simulink model "nonlinear_model_for_testing_params"  (R2016b)
settings: Solver=VariableStepAuto  StartTime=0.0  StopTime=20  RelTol=1e-3
values from neighbouring files (symbols this model uses):
  B_e = [[0 0] ... (first row only)    [init_heli_all.m]
  j_e = m_c*(l_c)^2 + 2*m_p*(l_h)^2    (= 1.033536)    [init_heli_all.m]
  j_lambda = m_c*(l_c)^2 + 2*m_p*((l_h)^2 + (l_p)^2)    (= 1.077636)    [init_heli_all.m]
  j_p = 2*m_p*(l_p)^2    (= 0.0441)    [init_heli_all.m]
  K = lqr(A, B, Q, R)    [init_heli_all.m]
  L = place(A_e',C_e',[-3,-4,-5,-7,-8,-10]).'    [init_heli_all.m]
  L1 = l_h*k_f    (= 0.10164)    [init_heli_all.m]
  L2 = k2*j_e    (= 0.10164)    [init_heli_all.m]
  L3 = l_h*k_f    (= 0.10164)    [init_heli_all.m]
  L4 = k_f*l_h*l_p    (= 0.017787)    [init_heli_all.m]
  P = inv(C*inv(B*K-A)*B)    [init_heli_all.m]
undefined symbols (not defined in the file or in its folder): A_est
settings Model: Creator=Kevin K. Kaldvansvik  LastModifiedBy=Kevin K. Kaldvansvik

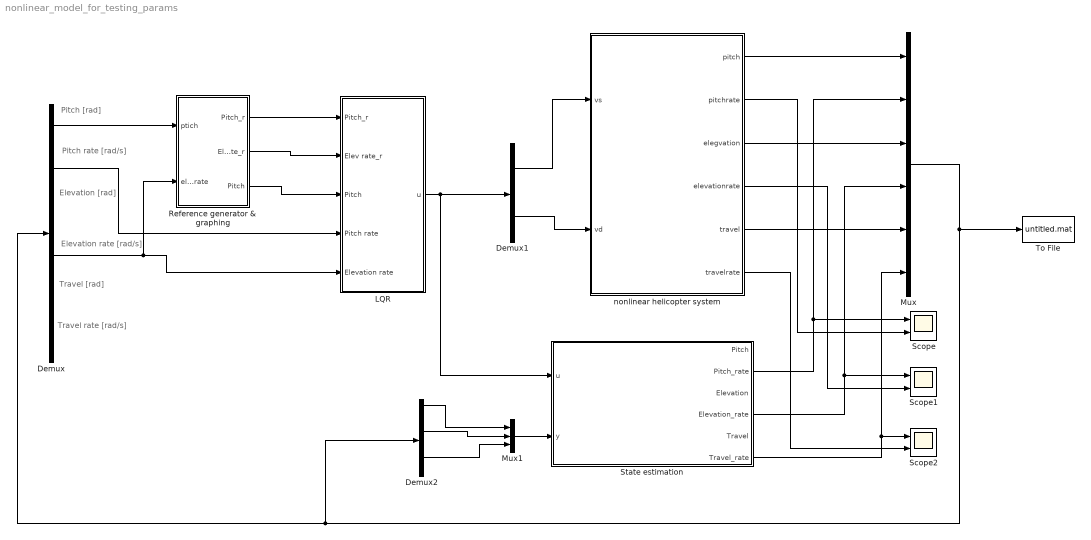
== system nonlinear_model_for_testing_params ==
  note: Travel rate [rad/s]
  note: Travel [rad]
  note: Elevation rate [rad/s]
  note: Elevation [rad]
  note: Pitch rate [rad/s]
  note: Pitch [rad]
  Demux : Demux  Outputs=6
  Demux1 : Demux  Outputs=2
  Demux2 : Demux  Outputs=6
  LQR : Subsystem
  Mux : Mux  Inputs=6
  Mux1 : Mux  Inputs=3
  Reference generator & graphing : Subsystem
  Scope : Scope  NumInputPorts=2
  Scope1 : Scope  NumInputPorts=2
  Scope2 : Scope  NumInputPorts=2
  State estimation : Subsystem
  To File : ToFile  MatrixName=kp_v1
  nonlinear helicopter system : Subsystem
  wires:
  Mux/1 -> Demux2/1, Demux/1, To File/1
  LQR/1(u) -> State estimation/1(u), Demux1/1
  Demux1/1 -> nonlinear helicopter system/1(vs)
  Demux1/2 -> nonlinear helicopter system/2(vd)
  Reference generator & graphing/1(Pitch_r) -> LQR/1(Pitch_r)
  Reference generator & graphing/2(Elevation_rate_r) -> LQR/2(Elev rate_r)
  Reference generator & graphing/3(Pitch) -> LQR/3(Pitch)
  nonlinear helicopter system/1(pitch) -> Mux/1
  nonlinear helicopter system/5(travel) -> Mux/5
  nonlinear helicopter system/3(elegvation) -> Mux/3
  State estimation/4(Elevation_rate) -> Scope1/1, Mux/4
  State estimation/6(Travel_rate) -> Scope2/1, Mux/6
  Demux/1 -> Reference generator & graphing/1(ptich)
  Demux/2 -> LQR/4(Pitch rate)
  Demux/4 -> Reference generator & graphing/2(elevrate), LQR/5(Elevation rate)
  Mux1/1 -> State estimation/2(y)
  Demux2/1 -> Mux1/1
  Demux2/3 -> Mux1/2
  Demux2/5 -> Mux1/3
  State estimation/2(Pitch_rate) -> Scope/1, Mux/2
  nonlinear helicopter system/2(pitchrate) -> Scope/2
  nonlinear helicopter system/4(elevationrate) -> Scope1/2
  nonlinear helicopter system/6(travelrate) -> Scope2/2

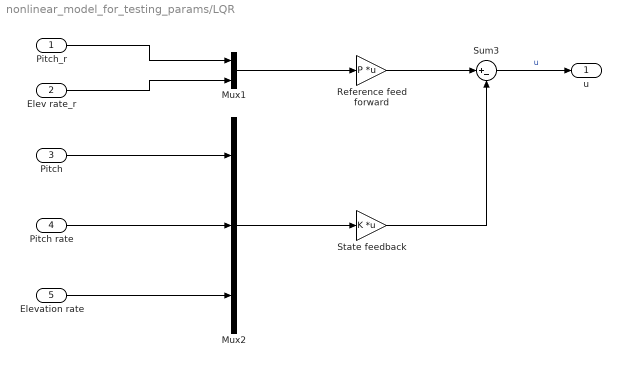
== system nonlinear_model_for_testing_params/LQR ==
  Pitch_r : Inport
  Elev rate_r : Inport  Port=2
  Pitch : Inport  Port=3
  Pitch rate : Inport  Port=4
  Elevation rate : Inport  Port=5
  Mux1 : Mux  Inputs=2
  Mux2 : Mux  Inputs=3
  "Reference feed forward " : Gain  Gain=P  Multiplication=Matrix(K*u)
  State feedback : Gain  Gain=K  Multiplication=Matrix(K*u)
  Sum3 : Sum  Inputs=|+-
  u : Outport
  wires:
  State feedback/1 -> Sum3/2
  "Reference feed forward "/1 -> Sum3/1
  Mux2/1 -> State feedback/1
  Mux1/1 -> "Reference feed forward "/1
  Sum3/1 -> u/1  "u"
  Elev rate_r/1 -> Mux1/2
  Pitch_r/1 -> Mux1/1
  Pitch/1 -> Mux2/1
  Pitch rate/1 -> Mux2/2
  Elevation rate/1 -> Mux2/3

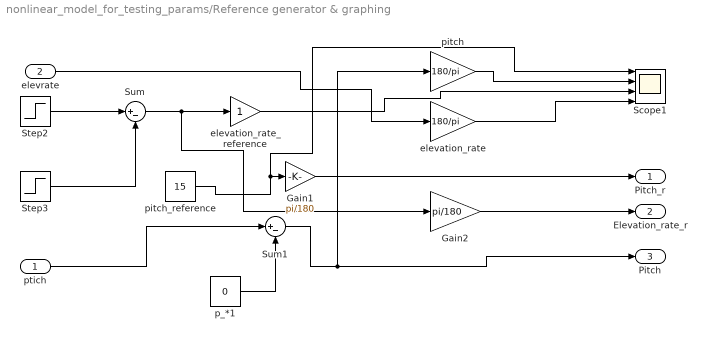
== system nonlinear_model_for_testing_params/Reference generator & graphing ==
  ptich : Inport
  elevrate : Inport  Port=2
  Gain1 : Gain  Gain=pi/180
  Gain2 : Gain  Gain=pi/180
  Scope1 : Scope  NumInputPorts=4
  Step2 : Step  After=5  SampleTime=0
  Step3 : Step  Time=4  After=5  SampleTime=0
  Sum : Sum  Inputs=|+-
  Sum1 : Sum  Inputs=|+-
  elevation_rate : Gain  Gain=180/pi
  elevation_rate_reference : Gain
  p_*1 : Constant  Value=0
  pitch : Gain  Gain=180/pi
  pitch_reference : Constant  Value=15
  Pitch_r : Outport
  Elevation_rate_r : Outport  Port=2
  Pitch : Outport  Port=3
  wires:
  Step3/1 -> Sum/2
  ptich/1 -> Sum1/1
  p_*1/1 -> Sum1/2
  Sum1/1 -> Pitch/1, pitch/1
  Step2/1 -> Sum/1
  Gain1/1 -> Pitch_r/1
  pitch_reference/1 -> Scope1/1, Gain1/1
  Sum/1 -> Gain2/1, elevation_rate_reference/1
  elevation_rate_reference/1 -> Scope1/3
  elevation_rate/1 -> Scope1/4
  pitch/1 -> Scope1/2
  Gain2/1 -> Elevation_rate_r/1
  elevrate/1 -> elevation_rate/1

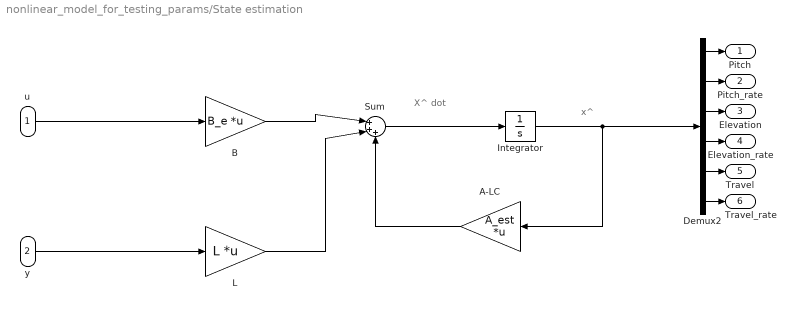
== system nonlinear_model_for_testing_params/State estimation ==
  note: x^
  note: X^ dot
  u : Inport
  y : Inport  Port=2
  A-LC : Gain  Gain=A_est  Multiplication=Matrix(K*u)
  B : Gain  Gain=B_e  Multiplication=Matrix(K*u)
  Demux2 : Demux  Outputs=6
  Integrator : Integrator
  L : Gain  Gain=L  Multiplication=Matrix(K*u)
  Sum : Sum  Inputs=|+++
  Pitch : Outport
  Pitch_rate : Outport  Port=2
  Elevation : Outport  Port=3
  Elevation_rate : Outport  Port=4
  Travel : Outport  Port=5
  Travel_rate : Outport  Port=6
  wires:
  B/1 -> Sum/1
  Sum/1 -> Integrator/1
  Integrator/1 -> A-LC/1, Demux2/1
  L/1 -> Sum/2
  A-LC/1 -> Sum/3
  Demux2/2 -> Pitch_rate/1
  Demux2/3 -> Elevation/1
  Demux2/4 -> Elevation_rate/1
  Demux2/5 -> Travel/1
  Demux2/1 -> Pitch/1
  u/1 -> B/1
  Demux2/6 -> Travel_rate/1
  y/1 -> L/1

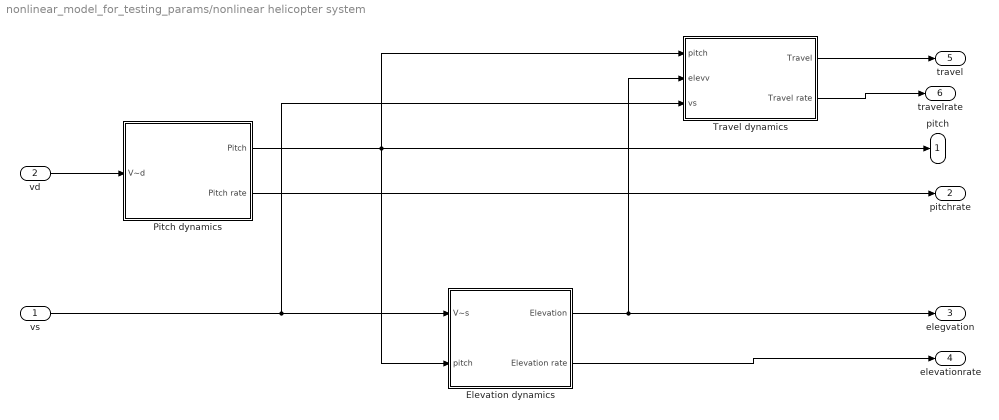
== system nonlinear_model_for_testing_params/nonlinear helicopter system ==
  vs : Inport
  vd : Inport  Port=2
  Elevation dynamics : Subsystem
  Pitch dynamics : Subsystem
  Travel dynamics : Subsystem
  pitch : Outport
  pitchrate : Outport  Port=2
  elegvation : Outport  Port=3
  elevationrate : Outport  Port=4
  travel : Outport  Port=5
  travelrate : Outport  Port=6
  wires:
  vd/1 -> Pitch dynamics/1(V~d)
  Elevation dynamics/1(Elevation) -> Travel dynamics/2(elevv), elegvation/1
  Pitch dynamics/2(Pitch rate) -> pitchrate/1
  vs/1 -> Elevation dynamics/1(V~s), Travel dynamics/3(vs)
  Pitch dynamics/1(Pitch) -> Elevation dynamics/2(pitch), Travel dynamics/1(pitch), pitch/1
  Travel dynamics/2(Travel rate) -> travelrate/1
  Travel dynamics/1(Travel) -> travel/1
  Elevation dynamics/2(Elevation rate) -> elevationrate/1

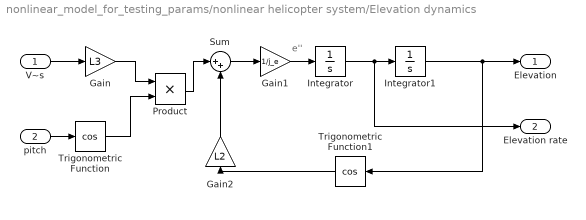
== system nonlinear_model_for_testing_params/nonlinear helicopter system/Elevation dynamics ==
  note: e''
  V~s : Inport
  pitch : Inport  Port=2
  Gain : Gain  Gain=L3
  Gain1 : Gain  Gain=1/j_e
  Gain2 : Gain  Gain=L2
  Integrator : Integrator
  Integrator1 : Integrator
  Product : Product
  Sum : Sum  Inputs=|++
  Trigonometric Function : Trigonometry  Operator=cos
  Trigonometric Function1 : Trigonometry  Operator=cos
  Elevation : Outport
  Elevation rate : Outport  Port=2
  wires:
  Integrator/1 -> Elevation rate/1, Integrator1/1
  V~s/1 -> Gain/1
  Integrator1/1 -> Trigonometric Function1/1, Elevation/1
  Gain/1 -> Product/1
  Sum/1 -> Gain1/1
  Gain1/1 -> Integrator/1
  Product/1 -> Sum/1
  pitch/1 -> Trigonometric Function/1
  Trigonometric Function/1 -> Product/2
  Trigonometric Function1/1 -> Gain2/1
  Gain2/1 -> Sum/2

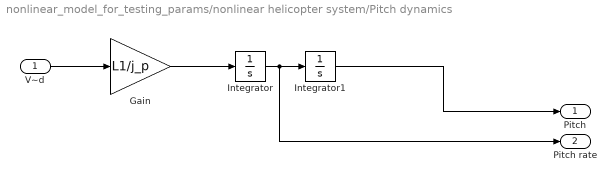
== system nonlinear_model_for_testing_params/nonlinear helicopter system/Pitch dynamics ==
  V~d : Inport
  Gain : Gain  Gain=L1/j_p
  Integrator : Integrator
  Integrator1 : Integrator
  Pitch : Outport
  Pitch rate : Outport  Port=2
  wires:
  Integrator/1 -> Pitch rate/1, Integrator1/1
  Integrator1/1 -> Pitch/1
  V~d/1 -> Gain/1
  Gain/1 -> Integrator/1

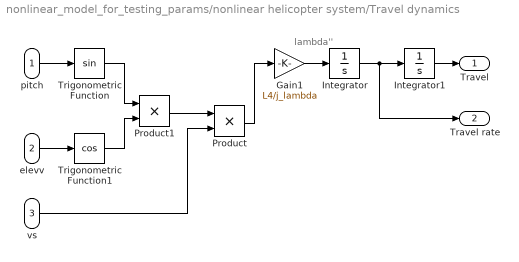
== system nonlinear_model_for_testing_params/nonlinear helicopter system/Travel dynamics ==
  note: lambda''
  pitch : Inport
  elevv : Inport  Port=2
  vs : Inport  Port=3
  Gain1 : Gain  Gain=L4/j_lambda
  Integrator : Integrator
  Integrator1 : Integrator
  Product : Product
  Product1 : Product
  Trigonometric Function : Trigonometry
  Trigonometric Function1 : Trigonometry  Operator=cos
  Travel : Outport
  Travel rate : Outport  Port=2
  wires:
  Integrator1/1 -> Travel/1
  Integrator/1 -> Integrator1/1, Travel rate/1
  pitch/1 -> Trigonometric Function/1
  Gain1/1 -> Integrator/1
  elevv/1 -> Trigonometric Function1/1
  Product/1 -> Gain1/1
  Trigonometric Function/1 -> Product1/1
  Trigonometric Function1/1 -> Product1/2
  vs/1 -> Product/2
  Product1/1 -> Product/1
